simulink subsystem "Data_processing"  (R2020a)
settings: Solver=VariableStepAuto  StartTime=0.0  StopTime=10.0  RelTol=1e-3
settings Model: Creator=decla  LastModifiedBy=decla

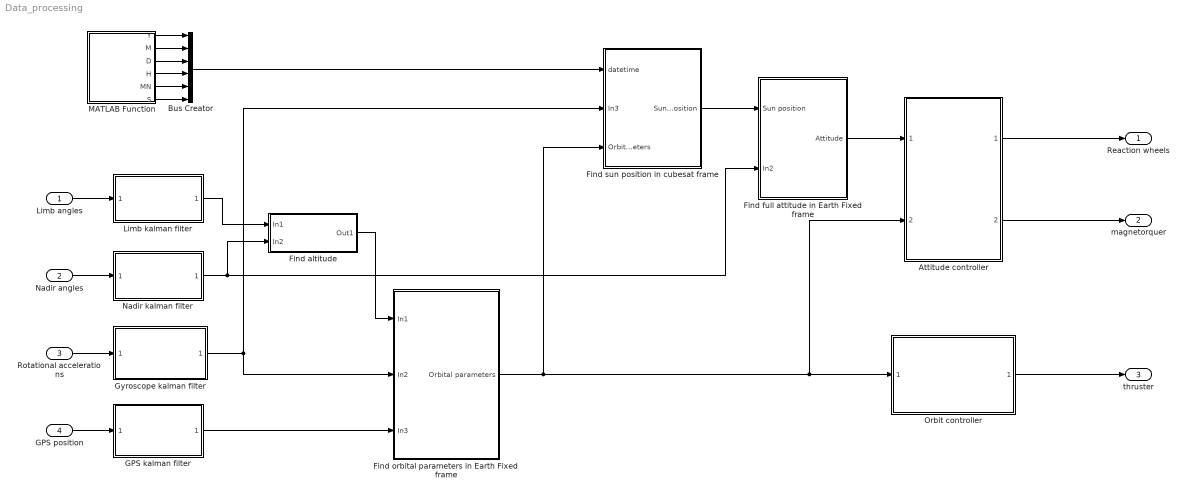
== system Data_processing ==
  Limb angles : Inport
  Nadir angles : Inport  Port=2
  Rotational accelerations : Inport  Port=3
  GPS position : Inport  Port=4
  Attitude controller : Subsystem  ReferencedSubsystem=Attitude_controller
  Bus Creator : BusCreator  Inputs=6
  Find altitude : Subsystem
  Find full attitude in Earth Fixed frame : Subsystem
  Find orbital parameters in Earth Fixed frame : Subsystem
  Find sun position in cubesat frame : Subsystem
  GPS kalman filter : Subsystem  ReferencedSubsystem=GPS_kalman_filter
  Gyroscope kalman filter : Subsystem  ReferencedSubsystem=Gyroscope_kalman_filter
  Limb kalman filter : Subsystem  ReferencedSubsystem=Limb_kalman_filter
  MATLAB Function : MATLAB Function  TreatAsAtomicUnit=on
  Nadir kalman filter : Subsystem  ReferencedSubsystem=Nadir_kalman_filter
  Orbit controller : Subsystem  ReferencedSubsystem=Orbit_controller
  Reaction wheels : Outport
  magnetorquer : Outport  Port=2
  thruster : Outport  Port=3
  wires:
  Limb angles/1 -> Limb kalman filter/1
  Nadir angles/1 -> Nadir kalman filter/1
  Rotational accelerations/1 -> Gyroscope kalman filter/1
  GPS position/1 -> GPS kalman filter/1
  Gyroscope kalman filter/1 -> Find sun position in cubesat frame/2(In3), Find orbital parameters in Earth Fixed frame/2(In2)
  GPS kalman filter/1 -> Find orbital parameters in Earth Fixed frame/3(In3)
  Find sun position in cubesat frame/1(Sun position) -> Find full attitude in Earth Fixed frame/1(Sun position)
  Find orbital parameters in Earth Fixed frame/1(Orbital parameters) -> Attitude controller/2, Orbit controller/1, Find sun position in cubesat frame/3(Orbital parameters)
  Orbit controller/1 -> thruster/1
  Attitude controller/1 -> Reaction wheels/1
  Attitude controller/2 -> magnetorquer/1
  Find full attitude in Earth Fixed frame/1(Attitude) -> Attitude controller/1
  MATLAB Function/1(Y) -> Bus Creator/1
  MATLAB Function/2(M) -> Bus Creator/2
  MATLAB Function/3(D) -> Bus Creator/3
  MATLAB Function/4(H) -> Bus Creator/4
  MATLAB Function/5(MN) -> Bus Creator/5
  MATLAB Function/6(S) -> Bus Creator/6
  Bus Creator/1 -> Find sun position in cubesat frame/1(datetime)
  Limb kalman filter/1 -> Find altitude/1(In1)
  Nadir kalman filter/1 -> Find altitude/2(In2), Find full attitude in Earth Fixed frame/2(In2)
  Find altitude/1(Out1) -> Find orbital parameters in Earth Fixed frame/1(In1)

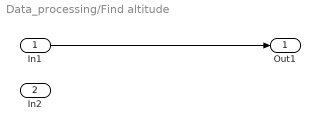
== system Data_processing/Find altitude ==
  In1 : Inport
  In2 : Inport  Port=2
  Out1 : Outport
  wires:
  In1/1 -> Out1/1

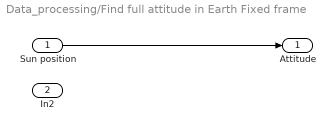
== system Data_processing/Find full attitude in Earth Fixed frame ==
  Sun position : Inport
  In2 : Inport  Port=2
  Attitude : Outport
  wires:
  Sun position/1 -> Attitude/1

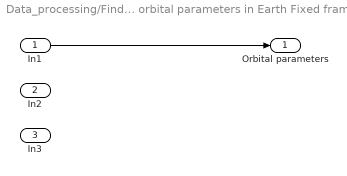
== system Data_processing/Find orbital parameters in Earth Fixed frame ==
  In1 : Inport
  In2 : Inport  Port=2
  In3 : Inport  Port=3
  Orbital parameters : Outport
  wires:
  In1/1 -> Orbital parameters/1

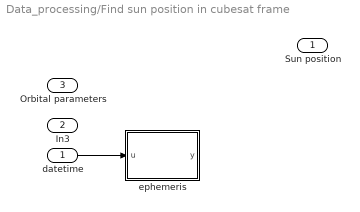
== system Data_processing/Find sun position in cubesat frame ==
  datetime : Inport
  In3 : Inport  Port=2
  Orbital parameters : Inport  Port=3
  ephemeris : MATLAB Function  TreatAsAtomicUnit=on
  Sun position : Outport
  wires:
  datetime/1 -> ephemeris/1(u)
  ? -> Sun position/1

== matlab function Data_processing/Find sun position in cubesat frame/ephemeris ==
  data: u input; y output
% https://ssd.jpl.nasa.gov/?planet_pos
function y = fcn(u)

y = u;

== matlab function Data_processing/MATLAB Function ==
  data: Y output; M output; D output; H output; MN output; S output
% https://www.mathworks.com/matlabcentral/answers/30479-how-to-get-system-date-and-time-into-simulink
function [Y, M, D, H, MN, S] = sysClock()
   coder.extrinsic('clock');
   Y = 0;
   M = 0;
   D = 0;
   H = 0;
   MN = 0;
   S = 0;
   [Y, M, D, H, MN, S] = clock;
end
